simulink model "Chap1_TimeVariantSystem"  (R2015a)
settings: Solver=ode45  StartTime=0.0  StopTime=1  RelTol=1e-3
PreLoadFcn:
  | Delay=[0 1/30.72e6 2/30.72e6 3/30.72e6 6/30.72e6 8/30.72e6];
  | Gain=[-3 0 -2 -6 -8 -10];
libraries: commchan3 x2, commrandsrc2 x1, commdigbbndam3 x1
settings Model: Creator=Larlyii-  LastModifiedBy=Administrator

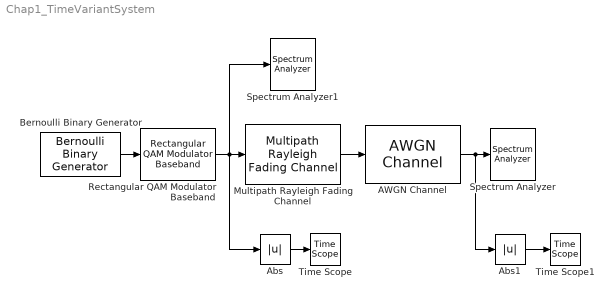
== system Chap1_TimeVariantSystem ==
  AWGN Channel : commchan3/AWGN Channel  InputProcessing=Columns as channels (frame based)  seed=67  noiseMode="Signal to noise ratio  (SNR)"  EbNodB=10  EsNodB=10  SNRdB=20  bitsPerSym=1  Ps=1  Tsym=1  variance=1
  Abs : Abs
  Abs1 : Abs
  Bernoulli Binary Generator : commrandsrc2/Bernoulli Binary Generator  P=0  seed=61  Ts=0.5e-3/(7*1200*4)  frameBased=on  sampPerFrame=7*1200*4  orient=off  outDataType=double
  Multipath Rayleigh Fading Channel : commchan3/Multipath Rayleigh Fading Channel  maxDopplerShift=40  spectrumType=Jakes  sigmaGaussian=1/sqrt(2)  coeffRounded=[1 -1.72 0.785]  freqMinMaxRJakes=[0 1]  freqMinMaxAJakes=[0 1]  sigmaGaussian1=1/sqrt(2)  sigmaGaussian2=1/sqrt(2)  centerFreqGaussian1=0.0  centerFreqGaussian2=0.0  gainGaussian1=0.5  gainGaussian2=0.5  coeffBell=9  dopplerSpectrum=doppler.jakes  pathDelays=Delay  avgPathGaindB=Gain  normalizePathGains=on  seed=73  enableProbe=0  openVisAtStart=off  outPathGains=off  outDelay=off
  Rectangular QAM Modulator Baseband : commdigbbndam3/Rectangular QAM Modulator Baseband  M=16  InType=Bit  Enc=Gray  Mapping=[0:15]  PowType=Average Power  MinDist=2  AvgPow=1  PeakPow=1  Ph=0  outDtype=double  outWordLen=16  outUDDataType=sfix(16)  outFracLenMode=Best precision  outFracLen=15
  Spectrum Analyzer : SpectrumAnalyzer
  Spectrum Analyzer1 : SpectrumAnalyzer
  Time Scope : TimeScope  DefaultConfigurationName=spbscopes.TimeScopeBlockCfg
  Time Scope1 : TimeScope  DefaultConfigurationName=spbscopes.TimeScopeBlockCfg
  wires:
  Bernoulli Binary Generator/1 -> Rectangular QAM Modulator Baseband/1
  Rectangular QAM Modulator Baseband/1 -> Spectrum Analyzer1/1, Abs/1, Multipath Rayleigh Fading Channel/1
  Multipath Rayleigh Fading Channel/1 -> AWGN Channel/1
  AWGN Channel/1 -> Abs1/1, Spectrum Analyzer/1
  Abs/1 -> Time Scope/1
  Abs1/1 -> Time Scope1/1
